simulink model "Simulation"  (R2022b)
settings: Solver=VariableStepAuto  StartTime=0.0  StopTime=0.1  RelTol=1e-3
undefined symbols (not defined in the file or in its folder): Ion, Lithium
libraries: spsDiodeLib x4, spsMosfetLib x4, spsSeriesRLCBranchLib x4, spsVoltageMeasurementLib x3, spsBatteryLib x1, spsCurrentMeasurementLib x1, spsDCVoltageSourceLib x1, spsLinearTransformerLib x1, spspowerguiLib x1
settings Model: Creator=Lenovo  LastModifiedBy=Lenovo

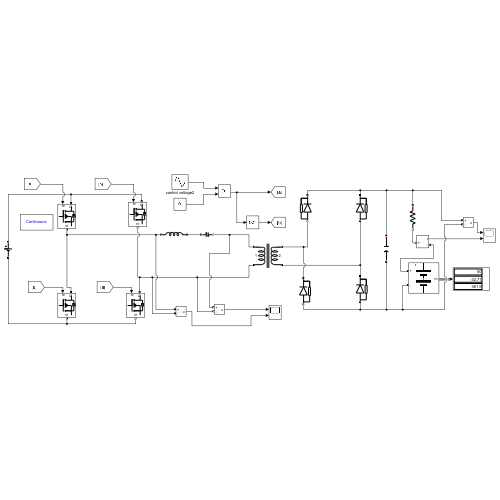
[thumbnail: Simulink's stored preview of the top-level diagram]
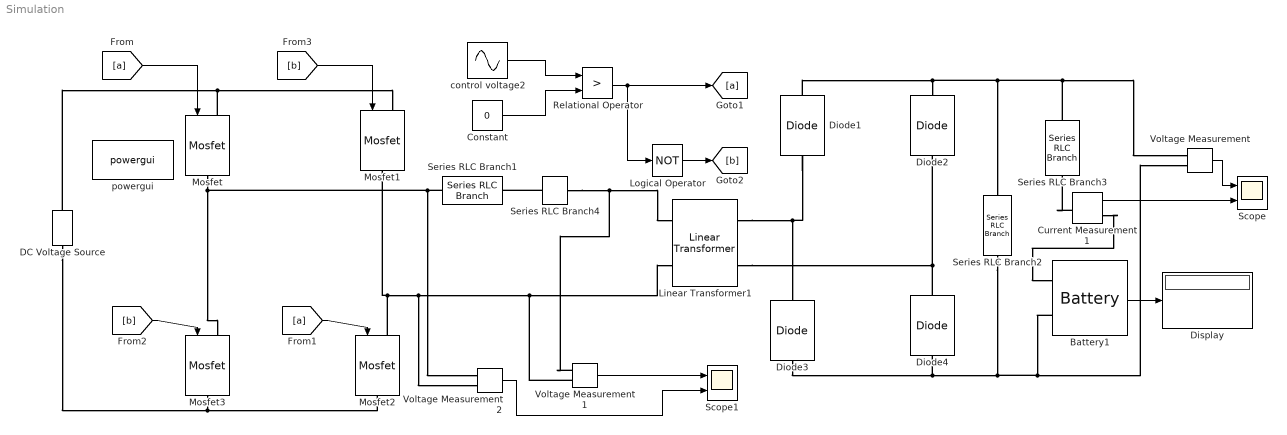
== system Simulation ==
  Battery1 : spsBatteryLib/Battery  BatType=Lithium-Ion  ShowTempParam=off  ThermalPreset=no  ShowAgeParam=off  NomV=335  NomQ=100  SOC=50  Batt_Tr=20  PresetModel=on  MaxQ=100  MinV=251.25  FullV=389.9357  Dis_rate=43.4783  R=0.0335  Normal_OP=90.4348  expZone="[361.9293      4.913043]"  current=[6.5 13 32.5]  Units=Time  Tci=20  NomT=20  T2=-30  MaxQ2=4.8  FullV2=7.1  Normal_OP2=5.655  expZone2="[6.58           1]"  Rca=0.6  ti=2000  Dp=0  Neq0=0  Tsim=1e6  Ta1=25  Qeol=5.4*0.9  Reol=0.013333*1.2  Char_age=[2.3478, 3]  Dis_age=[2.3478, 10]  N1=1500  N2=10500  N3=1000  N4=1400  Ta2=45  N5=950
  Constant : Constant  Value=0
  Current Measurement1 : spsCurrentMeasurementLib/Current Measurement  PhasorSimulation=off  OutputType=Complex  PSBequivalent=0
  DC Voltage Source : spsDCVoltageSourceLib/DC Voltage Source  Amplitude=400  Measurements=None
  Diode{1..4} (4 alike) : spsDiodeLib/Diode  Ron=0.001  Lon=0  Vf=0.8  IC=0  UseSnubber=0  Rs=500  Cs=250e-9  Measurements=off
  Display : Display
  Linear Transformer1 : spsLinearTransformerLib/Linear Transformer  UNITS=SI  NominalPower=[ 22e3 35e3 ]  winding1=[400 0 0]  winding2=[720 0 0]  ThreeWindings=off  winding3=[3.15e+05 0.7938 0.084225]  RmLm=[1e5 172e-6]  Measurements=Magnetization current  DataType=on
  Logical Operator : Logic  Operator=NOT  AllPortsSameDT=off  OutDataTypeStr=boolean
  Mosfet{,1..3} (4 alike) : spsMosfetLib/Mosfet  Ron=0.1  Lon=0  Rd=0.01  Vfd=0  IC=0  Rs=1e5  Cs=inf  Measurements=off
  Relational Operator : RelationalOperator  Operator=>  OutDataTypeStr=boolean  RndMeth=Simplest  InputSameDT=off
  Scope : Scope  NumInputPorts=2
  Scope1 : Scope  NumInputPorts=2
  Series RLC Branch1 : spsSeriesRLCBranchLib/Series RLC Branch  LConnTagsString=__new0  RConnTagsString=__new0  BranchType=L  Resistance=5  Inductance=34.4e-6  SetiL0=off  InitialCurrent=0  Capacitance=1e-6  Setx0=off  InitialVoltage=0  Measurements=None
  Series RLC Branch2 : spsSeriesRLCBranchLib/Series RLC Branch  LConnTagsString=__new0  RConnTagsString=__new0  BranchType=C  Resistance=5  Inductance=60e-6  SetiL0=off  InitialCurrent=0  Capacitance=60e-6  Setx0=off  InitialVoltage=0  Measurements=None
  Series RLC Branch3 : spsSeriesRLCBranchLib/Series RLC Branch  LConnTagsString=__new0  RConnTagsString=__new0  BranchType=R  Resistance=10  Inductance=1e-3  SetiL0=off  InitialCurrent=0  Capacitance=1e-6  Setx0=off  InitialVoltage=0  Measurements=None
  Series RLC Branch4 : spsSeriesRLCBranchLib/Series RLC Branch  LConnTagsString=__new0  RConnTagsString=__new0  BranchType=C  Resistance=5  Inductance=60e-6  SetiL0=off  InitialCurrent=0  Capacitance=0.6011e-6  Setx0=off  InitialVoltage=0  Measurements=Branch voltage
  Voltage Measurement : spsVoltageMeasurementLib/Voltage Measurement  PhasorSimulation=off  OutputType=Complex  PSBequivalent=0
  Voltage Measurement1 : spsVoltageMeasurementLib/Voltage Measurement  PhasorSimulation=off  OutputType=Complex  PSBequivalent=0
  Voltage Measurement2 : spsVoltageMeasurementLib/Voltage Measurement  PhasorSimulation=off  OutputType=Complex  PSBequivalent=0
  control voltage2 : Sin  Frequency=2*pi*35e3  SampleTime=0
  powergui : spspowerguiLib/powergui  Priority=1  SimulationMode=Continuous  SampleTime=50e-6  frequency=60  Iterations=50  frequencyindice=0  Pbase=100e6  ErrMax=1e-4  UnitsV=kV  UnitsW=MW  buscounter=0  FunctionMessages=off  echomessages=off  EnableUseOfTLC=off  CurrentSourceSwitches=off  DisableSnubberDevices=off  DisableRonSwitches=off  DisableVfSwitches=off  DisplayEquations=off  AutomaticDiscreteSolvers=off  SolverType=Tustin/Backward Euler (TBE)  Interpol=off  ExternalGateDelay=off  methode=off  Ts=100  x0status=blocks  SPID=on  SwTol=0  HookPort=off  NonlinearTolerance=1e-4  nMaxIteration=100  ContinueOnMaxIteration=off  RestoreLinks=warning  ResistiveCurrentMeasurement=off  Frange=[0:2:500]  Ylog=off  Xlog=on  ShowGrid=off  save=off  variable=ZData  structure=0  ZoomFFT=off  StartTime=0.0  cycles=1  DisplayStyle=1  fundamental=60  FreqAxis=off  MaxFrequency=1000  frequencyindicesteady=1  RmsSteady=1  display=off
  wires:
  [a] -> Mosfet/1
  [a] -> Mosfet2/1
  [b] -> Mosfet3/1
  [b] -> Mosfet1/1
  Voltage Measurement/1 -> Scope/1
  control voltage2/1 -> Relational Operator/1
  Constant/1 -> Relational Operator/2
  Relational Operator/1 -> [a], Logical Operator/1
  Logical Operator/1 -> [b]
  Current Measurement1/1 -> Scope/2
  Voltage Measurement1/1 -> Scope1/1
  Battery1/1 -> Display/1
  Voltage Measurement2/1 -> Scope1/2
  connections:
  Mosfet/LConn1 -- DC Voltage Source/RConn1 -- Mosfet1/LConn1
  Mosfet3/RConn1 -- DC Voltage Source/LConn1 -- Mosfet2/RConn1
  Diode1/LConn1 -- Linear Transformer1/RConn1 -- Diode3/RConn1
  Diode4/RConn1 -- Linear Transformer1/RConn2 -- Diode2/LConn1
  Series RLC Branch3/LConn1 -- Voltage Measurement/LConn1 -- Series RLC Branch2/LConn1 -- Diode2/RConn1 -- Diode1/RConn1
  Diode3/LConn1 -- Battery1/LConn2 -- Voltage Measurement/LConn2 -- Series RLC Branch2/RConn1 -- Diode4/LConn1
  Series RLC Branch4/LConn1 -- Voltage Measurement1/LConn1 -- Linear Transformer1/LConn1
  Mosfet2/LConn1 -- Voltage Measurement1/LConn2 -- Linear Transformer1/LConn2 -- Voltage Measurement2/LConn2 -- Mosfet1/RConn1
  Mosfet/RConn1 -- Voltage Measurement2/LConn1 -- Series RLC Branch1/RConn1 -- Mosfet3/LConn1
  Series RLC Branch4/RConn1 -- Series RLC Branch1/LConn1
  Current Measurement1/LConn1 -- Series RLC Branch3/RConn1
  Current Measurement1/RConn1 -- Battery1/LConn1
